simulink model "SLUGS2_UT"  (R2015a)
settings: Solver=FixedStepDiscrete  StartTime=0.0  StopTime=100  FixedStep=0.001  RelTol=1e-3
PreLoadFcn:
  | a=3;
  | Ts=0.01;
InitFcn:
  | a=3;
undefined symbols (not defined in the file or in its folder): A6, Pin, Timer
libraries: MCHP_Blockset x2, SLUGS_Library x1
settings Model: Creator=sharon  LastModifiedBy=sharon
settings OptimizationCC: InlineParams=on  InlineInvariantSignals=on  OptimizeModelRefInitCode=on  LifeSpan=1
settings HardwareCC: ProdBitPerInt=16  ProdBitPerPointer=16  ProdLargestAtomicInteger=Integer  ProdIntDivRoundTo=Zero  ProdEndianess=LittleEndian  ProdWordSize=16  ProdHWDeviceType=Generic->Custom
settings ModelReferenceCC: ModelReferenceNumInstancesAllowed=Single
settings RTWCC: SystemTargetFile=MCHP_dsPIC_stf.tlc  TemplateMakefile=MCHP_dsPIC.tmf  Description=Microchip Embedded Target PIC24 dsPIC30 dsPIC33 (real-time)
settings CodeAppCC: IgnoreCustomStorageClasses=off  MaxIdLength=255
settings STFCustomTargetCC: TargetLibSuffix=_lib.a  GenerateSampleERTMain=off  IncludeMdlTerminateFcn=off  CombineOutputUpdateFcns=on  SuppressErrorStatus=on  SupportContinuousTime=off  SupportNonInlinedSFcns=on  SupportVariableSizeSignals=off  SystemTargetFile=MCHP_dsPIC_stf.tlc
settings ERTTargetCC: TargetLibSuffix=_lib.a  GenerateSampleERTMain=off  IncludeMdlTerminateFcn=off  SuppressErrorStatus=on  SupportContinuousTime=off  SupportNonInlinedSFcns=on  SupportVariableSizeSignals=off  ERTSrcFileBannerTemplate=MCHP_dsPIC_code_template.cgt  ERTHdrFileBannerTemplate=MCHP_dsPIC_code_template.cgt  ERTDataSrcFileTemplate=MCHP_dsPIC_code_template.cgt  ERTDataHdrFileTemplate=MCHP_dsPIC_code_template.cgt  ERTCustomFileTemplate=MCHP_main.tlc

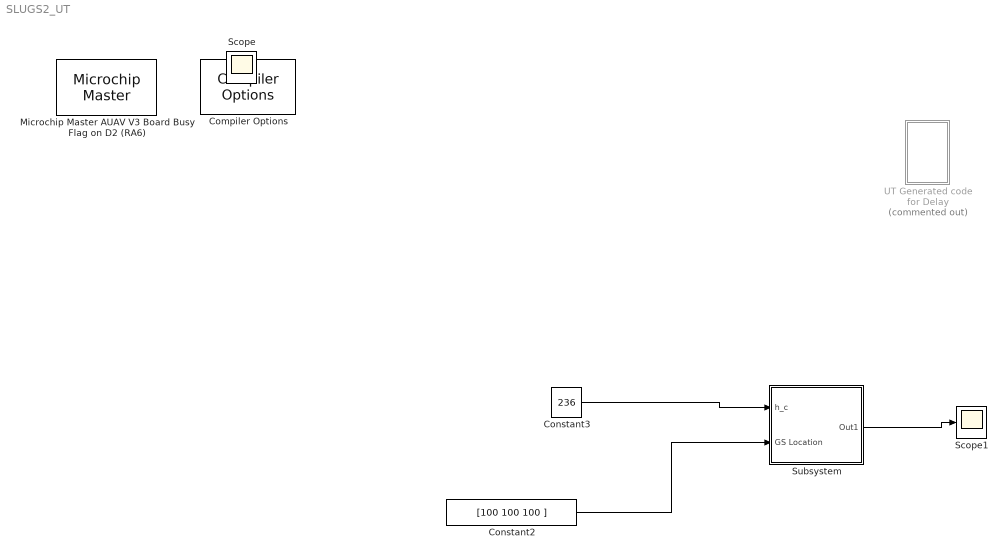
== system SLUGS2_UT ==
  Compiler Options : MCHP_Blockset/System Configuration/Compiler Options  Priority=1  LATEST_CMPLR=on  COMP_LIST=Dynamic Options  COMP_LIST_TXT=xc16 - v1.26  USE_64BIT_DOUBLE=off  MCHP_MULTITHREAD_COMPILATION=on  MCHP_MASTERLINK=|  OPTIMIZATION_LEVEL=1  MPLAB_LINKLIB=default  MPLAB_LINKLIB1=default  UNROLL_LOOPS=off  OMIT_FRAME_POINTER=off  PROCEDURAL_ABSTRACTION=off  MCONST=in code memory  MDATA=Can use all available memory  MSCALAR=Can use all available memory  MCODE=is more than 32768  HEAP_SIZE=0  OMF=elf  DEBUG_INFO=off  AssemblyListing=on  ProduceHexOutput=on
      | SLUGS2_UT/Microchip Master
      | AUAV V3 Board
      | Busy Flag on D2 (RA6)
  Constant2 : Constant  Value=[100 100 100 ]  OutDataTypeStr=single  SampleTime=-1
  Constant3 : Constant  Value=236  OutDataTypeStr=single  SampleTime=-1
  Microchip Master AUAV V3 Board Busy Flag on D2 (RA6) : MCHP_Blockset/System Configuration/Microchip Master  Priority=1  PICREF=33EP512MU810  TIMESTEP_REF="Timer  ( 0.001s )"  BUSYFLAG=Dynamic Options  BUSYFLAG_TXT=A6 / Pin[91]  PWRTEN=PWRT enabled  BOREN=Disable  BODENV=2.7V  BORV=Brown-out Reset set at 2.0V  FPWRT=128ms  DSBOREN=Deep Sleep BOR enabled in Deep Sleep  DSLPBOR=Deep Sleep BOR enabled in Deep Sleep  MCLRE=Enabled  SMCLR=MCLR pin generates a normal system Reset  PMDL1WAY=Allow only one reconfiguration  RSTPRI=Device will obtain reset instruction from Primary flash  TEMP=Not used  SOSCSRC=Analog Mode for use with crystal  SOSCSEL=Secondary oscillator configured for high-power operation  IOL1WAY=Allow only one reconfiguration  ALTVREF=Voltage reference input; ADC =RA9/RA10 Comparator =RA9;RA10  DISUVREG=Regulator is disabled  DSSWEN=Deep Sleep is controlled by the register bit DSEN  LPCFG=Disabled - regardless of RETEN  RTCBAT=RTC operation is continued through VBAT  VBTBOR=VBAT BOR enabled  WUTSEL=Default regulator start-up time used  POWERSAVE=off  FNOSC=Primary oscillator (XT; HS; EC)  FPR=ECIO w/ PLL 16x  FOSFPR=HS3 w/PLL 16x  FOS=Internal Fast RC  FRANGE=High Range  OSCILLATOR_SELECT=Crystal / Ceramic resonator  OSCILLATOR_SELECT_spd=Crystal / Ceramic resonator  QUARTZ=8e6  QUARTZ_spd=8e6  POSCGAIN=2x gain setting  POSCBOOST=Boost the kick start of the oscillator  SOSCGAIN=2x gain setting  SOSCBOOST=Boost the kick start of the oscillator  ACTIV_PLL=on  ACTIV_PLL_spd=on  MIPS_DESIRED=70e6  MIPS_DESIRED_spd=70e6  FPLLMUL=24x Multiplier  FPLLIDIV=8x Divider  POSCFREQ=Primary oscillator/external clock input frequency greater than 8MHz  POSCMD=XT Crystal Oscillator Mode  POSCMOD=Primary Oscillator Disabled  MIPS=70 * 1e6  FPLLODIV=32x Divider  PLLKEN=Clock switch to PLL source will wait until the PLL lock signal is valid.  FCKSM=Both Clock Switching and Fail-safe Clock Monitor are enabled  FCKSMEN=Sw Disabled; Mon Disabled  IESO=Start up with FRC; then switch  DSWDTPS=1:2;147;483;648 (25.7 Days)  FWDTEN=Disable  FWDTWINSZ=Window size is 25%  FWPSA=1:512  FWPSA0=1:128  FWPSB=1:16  WDT=Disable  WDTPOST=1:32768  WDTPRE=1:128  WDTPS=1:32768  WINDIS=Watchdog Timer in Non-Window mode  WWDTEN=Non-Window mode  DSWDTEN=DSWDT enabled  DSWDTOSC=DSWDT uses Low Power RC Oscillator (LPRC)  FPBDIV=Pb_Clk is Sys_Clk/8  FSOSCEN=Enable SOSC  LPRCSEL=High Power; High Accuracy Mode  OSCIOFCN=OSCO/CLKO/RC15 functions as CLKO (FOSC/2)  OSCIOFNC=OSC2 is general purpose digital I/O pin  LVRCFG=Low Voltage regulator is not available  PLL_96MHZ=Enabled  PLL96MHZ=96 MHz PLL Startup is enabled automatically on start-up  PLLDIV=PLL is disabled  WDTCLK=WDT uses LPRC  WDTCMX=WDT clock source is determined by the WDTCLK Configuration bits  WDTWIN=WDT Window is 25% of WDT period  APL=Aux Flash Code protect is disabled  APLK=Aux Flash Write Protection and Code Protection is Disabled  AWRP=Auxiliary program memory is not write-protected  BSS=No boot program Flash segment  BWP=Protection Disabled  BWRP=Boot Segment may be written  CP=Protection Disabled  EBS=No Boot EEPROM  ESS=No Segment Data EEPROM  GCP=Disable  GSS=General Segment Code protect is disabled  GSS0=No protection  GSSK=General Segment Write Protection and Code Protection is Disabled  GWRP=General Segment may be written  PWP=Disable  RBS=No Boot RAM  RSS=No Secure RAM  SSS=No Secure Segment  SWRP=Secure segment may be written  WPCFG=Disable  WPDIS=Disable  WPEND=Write Protect from WPFP to the last page of memory  WPFP=Page 127 (0x1FC00)  ICESEL=Communicate on PGEC1/PGED1  ICS=Communicate on PGEC3 and PGED3  JTAGEN=Disable  COE=Reset Into Operational Mode  RES=Not used  DEBUG=Debugger is disabled  BACKBUG=Not used  BKBUG=Device resets into Operational mode  ALTI2C=I2C mapped to SDA1/SCL1 pins  ALTI2C1=SDA1/SCK1 pins are selected as the I/O pins for I2C1  ALTI2C2=SDA2/SCK2 pins are selected as the I/O pins for I2C2  ALTQIO=QEA1; QEB1; INDX1 are selected as inputs to QEI1  ALTSS1=SS1A is selected as the I/O pin for SPI1  CMPPOL0=Hysteresis is applied to falling edge  CMPPOL1=Hysteresis is applied to falling edge  FCANIO=Default CAN I/O  FETHIO=Default Ethernet I/O  FMIIEN=MII Enabled  FSRSSEL=SRS Priority 7  FUSBIDIO=Controlled by the USB Module  FVBUSONIO=Controlled by USB Module  HPOL=Active High  HYST0=45 mV Hysteresis  HYST1=45 mV Hysteresis  I2C1SEL=Use Default SCL1/SDA1 Pins For I2C1  LPOL=Active High  PWMPIN=Control with PORT/TRIS regs  RTCOSC=RTCC uses Secondary Oscillator (SOSC)  UPLLEN=USB PLL is enabled  UPLLIDIV=12x Divider  ATMOD8=Not used  ALTPMP=EPMP pins are in default location mode  I2C2SEL=I2C2 is multiplexed to SDA2/RA3 and SCL2/RA2  ALTADREF=AVREF+/AVREF- are mapped to RA9/RA10  ALTCVREF=CVREF+/CVREF- are mapped to RA9/RA10  PWMLOCK=PWM registers may be written without key sequence  MCHP_TIMER_REQUEST={Time Step}{TS}0:2:3:1:[]:70000;  MCHP_TIMER_RESULT=[1 8748.9999999999927 ]  MCHP_PORT={Busy Flag}{Busy}0:1:A6;  MCHP_PLLRegisters="[5    243  16385     -1]"  MCHPVAR=MCHP.fcy.periph=70000000;MCHP.fcy.MIPS=70000000;MCHP.PowerSave=0;MCHP.TimeStepFactor=MCHP_Fun.Hex2num('[3FF0000000000004]');MCHP.TimeStep_Timer=1;MCHP.NTIMERS=9;MCHP.id.name='33EP512MU810';MCHP.id.N=reshape([33 512 810],1,3);MCHP.id.L=reshape({ 'EP','MU',''},1,3);MCHP.id.Arch=3;MCHP.periph.PPS.reg_RPINRx=reshape([-1 1 1 1 1 -1 1 1 1 1 1 1 1 1 1 1 1 1 1 1 1 1 -1 -1 1 1 1 1 1 1 1 1 1 1 1 1 1 1 1 1 1 1 1 -1 -1 -1 1 -1 -1 -1 -1 -1 1 1 1 1 1 1 1 1 1 -1 1 1 1 -1 1 1 1 1 1 1 1 1 -1 1 1 1 1 1 1 1 1 -1 1 1 1],1,87);MCHP.PPS.dsPIC.RP=reshape([-1 -1 -1 -1 -1 -1 -1 -1 -1 -1 -1 -1 -1 -1 -1 -1 -1 -1 -1 -1 -1 -1 -1 -1 -1 -1 -1 -1 -1 -1 -1 -1 -1 -1 -1 -1 -1 -1 -1 -1 -1 -1 -1 -1 -1 -1 -1 -1 -1 -1 -1 -1 -1 -1 -1 -1 -1 -1 -1 -1 -1 -1 -1 -1 48 49 50 51 52 53 54 55 -1 -1 -1 -1 -1 -1 -1 63 64 -1 66 -1 68 69 -1 71 -1 -1 -1 -1 -1 -1 -1 -1 80 81 82 83 84 85 -1 -1 88 -1 -1 -1 92 93 -1 -1 96 97 -1 -1 -1 -1 102 -1 104 -1 -1 -1 -1 109 110 111],1,128);MCHP.PPS.dsPIC.RPI=reshape([-1 -1 -1 -1 -1 -1 -1 -1 -1 -1 -1 -1 -1 -1 -1 -1 0 1 2 3 4 5 6 7 -1 -1 -1 -1 -1 -1 14 15 16 17 18 19 20 21 22 23 24 25 26 27 28 29 30 31 -1 33 34 35 36 -1 -1 -1 -1 -1 -1 -1 44 45 46 -1 -1 -1 -1 -1 -1 -1 -1 -1 56 57 58 59 60 61 62 -1 -1 65 -1 67 -1 -1 70 -1 72 73 -1 -1 -1 -1 -1 -1 -1 -1 -1 -1 -1 -1 -1 -1 -1 -1 -1 -1 -1 -1 -1 -1 -1 -1 -1 -1 -1 -1 -1 103 -1 105 -1 -1 108],1,125);MCHP.PPS.dsPIC.RPINR_list=reshape({ '1','INT1','INT2','INT3','INT4','T1CK','T2CK','T3CK','T4CK','T5CK','T6CK','T7CK','T8CK','T9CK','IC1','IC2','IC3','IC4','IC5','IC6','IC7','IC8','OCFA','OCFB','FLT1','FLT2','FLT3','FLT4','QEA1','QEB1','INDX1','HOME1','QEA2','QEB2','INDX2','HOME2','U1RX','U1CTS','U2RX','U2CTS','SDI1','SCK1','SS1','44','SDI2','SCK2','SS2','48','CSDIR','CSCK','COFS','52','C1RX','C2RX','U3RX','U3CTS','U4RX','U4CTS','SDI3','SCK3','SS3','62','SDI4','SCK4','SS4','66','IC9','IC10','IC11','IC12','IC13','IC14','IC15','IC16','OCFC','SYNCI1','SYNCI2','DTCMP1','DTCMP2','DTCMP3','DTCMP4','DTCMP5','DTCMP6','DTCMP7','FLT5','FLT6','FLT7','FLT8','89','SENT1','SENT2','92'},1,92);MCHP.PPS.dsPIC.RPOR_list=reshape({ '1','U1TX','U1RTS','U2TX','U2RTS','SDO1','SCK1','SS1','SDO2','SCK2','SS2','CSDO','CSCK','COFS','C1TX','C2TX','OC1','OC2','OC3','OC4','OC5','OC6','OC7','OC8','C1OUT','C2OUT','C3OUT','U3TX','U3RTS','U4TX','U4RTS','SDO3','SCK3','SS3','SDO4','SCK4','SS4','OC9','OC10','OC11','OC12','OC13','OC14','OC15','OC16','SYNCO1','SYNCO2','QEI1CCMP','QEI2CCMP','REFCLK','C4OUT','C5OUT','52','53','54','55','56','SENT1','SENT2'},1,59);MCHP.PPS.map_RPnR_RPORx=reshape([64 65 66 67 68 69 70 71 79 80 82 84 85 87 96 97 98 99 100 101 -1 -1 104 108 109 112 113 118 120 125 126 127],1,32);MCHP.Rx=reshape([17 25 -1 72 93 87 90 -1 -1 -1 -1 38 24 6 76 94 88 89 -1 -1 -1 -1 58 23 7 77 98 52 57 -1 -1 -1 -1 59 22 8 78 99 51 56 -1 -1 -1 -1 60 21 9 81 100 49 -1 -1 -1 -1 -1 61 20 -1 82 3 50 -1 -1 -1 -1 -1 91 26 -1 83 4 -1 10 -1 -1 -1 -1 92 27 -1 84 5 -1 11 -1 -1 -1 -1 -1 32 -1 68 18 53 12 -1 -1 -1 -1 28 33 -1 69 19 -1 14 -1 -1 -1 -1 29 34 -1 70 -1 -1 -1 -1 -1 -1 -1 -1 35 -1 71 -1 -1 -1 -1 -1 -1 -1 -1 41 63 79 -1 40 96 -1 -1 -1 -1 -1 42 73 80 -1 39 97 -1 -1 -1 -1 66 43 74 47 -1 -1 95 -1 -1 -1 -1 67 44 64 48 -1 -1 1 -1 -1 -1 -1],11,16);MCHP.ADC.ANtype=reshape([3 1],1,2);MCHP.ADC.ADCONx=reshape([47103 59391 40959 263 0 0],1,6);MCHP.ADC.ADCHS_0=reshape([40863 1799],1,2);MCHP.ADC.Flags=reshape([1 0],1,2);MCHP.ADC.Buffer=reshape([16 16],1,2);MCHP.ADC.port=reshape([16 17 18 19 20 21 22 23 24 25 26 27 28 29 30 31 33 34 35 36 72 73 6 7 64 65 66 67 68 69 70 71 -1 -1 -1 -1 -1 -1 -1 -1 -1 -1 -1 -1 -1 -1 -1 -1 -1 -1 -1 -1 -1 -1 -1 -1 -1],1,57);MCHP.ADC.port_VrefP=-1;MCHP.ADC.port_VrefM=-1;MCHP.ADC.port_AVdd=-1;MCHP.ADC.port_AVss=-1;MCHP.memory.RAM=53248;MCHP.memory.RAM_XBegin=4096;MCHP.memory.RAM_YBegin=36864;MCHP.memory.RAM_dma=reshape([53248 57344],1,2);MCHP.DMA.Num=15;MCHP.DMA.CNTmax=16383;MCHP.QEI.QEICONx=reshape([49023 49023 -1 -1 -1 -1],1,6);MCHP.QEI.QEItype=2;MCHP.QEI.Port_QEI_INDX=reshape([-1 -1],1,2);MCHP.QEI.Port_QEI_QEA=reshape([-1 -1],1,2);MCHP.QEI.Port_QEI_QEB=reshape([-1 -1],1,2);MCHP.QEI.Port_QEI_UPDN=reshape([-1 -1],1,2);MCHP.INT.Port=reshape([48 32767 32767 32767 32767],1,5);MCHP.PWM_HS.Flags=reshape([6 2 1],1,3);MCHP.PWM.port_FLT=reshape([-1 -1 -1 -1 -1 -1 -1 -1 -1 -1 -1 -1 -1 -1 -1 -1 -1 -1 -1 -1 -1 -1 -1 -1 -1 -1 -1 -1 -1 -1 -1 -1 -1],1,33);MCHP.PWM.PWMRef=-1;MCHP.PWM.Flag=0;MCHP.PWM.Port_PWM_l=reshape([64 -1 66 -1 68 -1 70 -1 33 -1 35 -1 -1 -1 -1 -1 -1 -1],2,9);MCHP.PWM.Port_PWM_h=reshape([65 -1 67 -1 69 -1 71 -1 34 -1 36 -1 -1 -1 -1 -1 -1 -1],2,9);MCHP.IC.Port=reshape([32767 32767 32767 32767 32767 32767 32767 32767 32767 32767 32767 32767 32767 32767 32767 32767],1,16);MCHP.IC.type=1;MCHP.OC.Port=reshape([32767 32767 32767 32767 32767 32767 32767 32767 32767 32767 32767 32767 32767 32767 32767 32767],1,16);MCHP.OC.type=1;MCHP.CN.Port=reshape([-1 -1 -1 -1 -1 -1 -1 -1 -1 -1 -1 -1 -1 -1 -1 -1 -1 -1 -1 -1 -1 -1 -1 -1 -1 -1 -1 -1 -1 -1 -1 -1 -1 -1 -1 -1 -1 -1 -1 -1 -1 -1 -1 -1 -1 -1 -1 -1 -1 -1 -1 -1 -1 -1 -1 -1 -1 -1 -1 -1 -1 -1 -1 -1 -1 -1 -1 -1 -1 -1 -1 -1 -1 -1 -1 -1 -1 -1 -1 -1 -1 -1 -1 -1 -1],1,85);MCHP.CN.PullUp=reshape([50943 65535 61470 65535 1023 12607 62403 0 0 0 0],1,11);MCHP.CN.type=1;MCHP.CN.Flag_PullDown=1;MCHP.SPI.Refs=reshape([1 2 3 4 0 0],1,6);MCHP.SPI.SPIxCON1=8191;MCHP.SPI.SPIxCON2=57347;MCHP.SPI.Port_SDI=reshape([-1 103 -1 -1 -1 -1],1,6);MCHP.SPI.Port_SDO=reshape([-1 104 -1 -1 -1 -1],1,6);MCHP.SPI.Port_SCK=reshape([-1 102 -1 -1 -1 -1],1,6);MCHP.SPI.Port_SS=reshape([-1 -1 -1 -1 -1 -1],1,6);MCHP.I2C.Refs=reshape([1 2 0 0 0],1,5);MCHP.I2C.I2CxCON=49151;MCHP.I2C.NewRegName=1;MCHP.I2C.Port_SDA=reshape([-1 84 -1 -1 -1],1,5);MCHP.I2C.Port_SCL=reshape([-1 85 -1 -1 -1],1,5);MCHP.I2C.Port_ASDA=reshape([57 3 -1 -1 -1],1,5);MCHP.I2C.Port_ASCL=reshape([58 2 -1 -1 -1],1,5);MCHP.I2C.Fuse_Port_SCL_SDA=reshape([17 1 18 1 -1 -1 -1 -1 -1 -1],2,5);MCHP.I2C.Fuse_Port_ASCL_ASDA=reshape([17 2 18 2 -1 -1 -1 -1 -1 -1],2,5);MCHP.Comp.Port_CVrefin=-1;MCHP.Comp.Port_CVref=26;MCHP.Comp.Port_CVref1O=-1;MCHP.Comp.Port_CVref2O=-1;MCHP.Comp.Port_CxOUT=reshape([32767 32767 32767 -1 -1],1,5);MCHP.Comp.Port_OAxOUT=reshape([-1 -1 -1 -1 -1],1,5);MCHP.Comp.Port_CxINP=reshape([21 19 55 -1 -1],1,5);MCHP.Comp.Port_CxINM=reshape([103 20 102 -1 105 18 104 -1 46 54 45 -1 -1 -1 -1 -1 -1 -1 -1 -1],4,5);MCHP.Comp.nComp=reshape([3 0 0],1,3);MCHP.Comp.OpAmp=0;MCHP.Comp.CVRCON=reshape([2047 0],1,2);MCHP.UART.port_Rx=reshape([32767 32767 32767 32767 -1 -1],1,6);MCHP.UART.port_Tx=reshape([32767 32767 32767 32767 -1 -1],1,6);MCHP.UART.port_ARx=reshape([-1 -1],1,2);MCHP.UART.port_ATx=reshape([-1 -1],1,2);MCHP.UART.port_RTS=reshape([32767 32767 32767 32767 -1 -1],1,6);MCHP.UART.port_CTS=reshape([32767 32767 32767 32767 -1 -1],1,6);MCHP.UART.reg_UxMODE=reshape([48127 48127 48127 48127 -1 -1],1,6);MCHP.UART.reg_UxSTA=reshape([61439 61439 61439 61439 -1 -1],1,6);  MCHP_CRC=2006118  BTMODE=Device is in Single Boot (legacy) mode  RES1=Not used  PLLSS=PLL is fed by the Primary oscillator  RES2=Not used  ALTCMPI=C1INC is on RB13; C2INC is on RB9 and C3INC is on RA0  BOREN1=BOR Enabled [When BOREN=1]  ALTRB6=Append the RP6/ASCL1/PMPD6 functions of RB6 to RA1 pin functions  RETCFG=Retention regulator is not available  DFMCY=Not used  BSS2=No Boot Segment  BSEN=No Boot Segment  CWRP=Configuration Segment may be written  CSS=No Protection (other than CWRP)  AIVTDIS=Disabled AIVT  BSLIM=Not used  WDTEN=Disable  BTSWP=Not used  DBCC=Not used  CTXT1=Not Assigned  CTXT2=Not Assigned  SEQNUM=Not used  nSEQNUM=Not used  BOREN0=Enabled  DMTIVT=Not used  DMTCNT=2^31 (2147483648)  DMTEN=Dead Man Timer is Enabled and cannot be disabled by software  ON=Not used  USERID=Not used  RESERVED1=Not used  PGL1WAY=Allow only one reconfiguration  FPLLRNG=34-68 MHz Input  FPLLICLK=FRC is input to the System PLL  FPLLMULT=PLL Multiply by 128  UPLLFSEL=USB PLL input is 24 MHz  DMTINTV=Window/Interval value is 127/128 counter value  WDTSPGM=WDT stops during Flash programming  FDMTEN=Deadman Timer is disabled  TRCEN=Trace features in the CPU are enabled  BOOTISA=Boot code and Exception code is MIPS32  FECCCON=ECC and Dynamic ECC are disabled (ECCCON bits are writable)  EXTDDRSIZE=External DDR2 Size is 128 MB  FSLEEP=Flash is powered down when the device is in Sleep mode  DBGPER=Allow CPU access to all permission regions  EJTAGBEN=Normal EJTAG functionality  TSEQ=Not used  CSEQ=Not used
  Scope1 : Scope
  Subsystem : Subsystem
  UT Generated code for Delay : Subsystem  Commented=on
  Scope : Scope
  wires:
  Constant3/1 -> Subsystem/1(h_c)
  Constant2/1 -> Subsystem/2(GS Location)
  Subsystem/1(Out1) -> Scope1/1

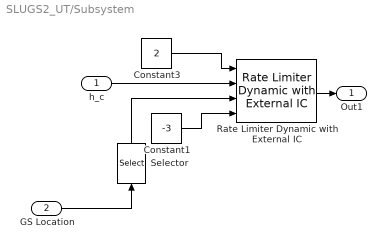
== system SLUGS2_UT/Subsystem ==
  h_c : Inport
  GS Location : Inport  Port=2
  Constant1 : Constant  Value=-3  OutDataTypeStr=single  SampleTime=-1
  Constant3 : Constant  Value=2  OutDataTypeStr=single  SampleTime=-1
  Rate Limiter Dynamic with External IC : SLUGS_Library/Singnal Routing & Conditioning/Rate Limiter Dynamic with External IC  rlIC=-1
  Selector : Selector  InputPortWidth=3  Indices=[1 ]
  Out1 : Outport
  wires:
  Rate Limiter Dynamic with External IC/1 -> Out1/1
  Constant1/1 -> Rate Limiter Dynamic with External IC/4
  h_c/1 -> Rate Limiter Dynamic with External IC/2
  Selector/1 -> Rate Limiter Dynamic with External IC/3
  GS Location/1 -> Selector/1
  Constant3/1 -> Rate Limiter Dynamic with External IC/1

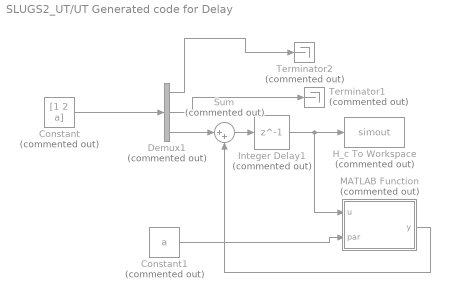
== system SLUGS2_UT/UT Generated code for Delay ==
  Constant : Constant  Commented=on  Value=[1 2 a]
  Constant1 : Constant  Commented=on  Value=a
  Demux1 : Demux  Commented=on  Outputs=3
  H_c To Workspace : ToWorkspace  Commented=on  VariableName=simout  SaveFormat=Timeseries  SampleTime=-1
  Integer Delay1 : Delay  Commented=on  DelayLength=1  InitialCondition=100  InputProcessing=Inherited  SampleTime=1
  MATLAB Function : MATLAB Function  Commented=on  TreatAsAtomicUnit=on
  Sum : Sum  Commented=on  Inputs=|++
  Terminator1 : Terminator  Commented=on
  Terminator2 : Terminator  Commented=on
  wires:
  Demux1/3 -> Sum/1
  Constant/1 -> Demux1/1
  Demux1/1 -> Terminator2/1
  Sum/1 -> Integer Delay1/1
  Constant1/1 -> MATLAB Function/2(par)
  Demux1/2 -> Terminator1/1
  Integer Delay1/1 -> MATLAB Function/1(u), H_c To Workspace/1
  MATLAB Function/1(y) -> Sum/2

== matlab function SLUGS2_UT/UT Generated code for Delay/MATLAB Function ==
  data: u input; y output; par input
function y = fcn(u,par)
%#codegen

y = u+par;
